simulink model "simulink_control"  (R2020b)
settings: Solver=FixedStepAuto  StartTime=0.0  StopTime=UI.motion_duration  FixedStep=UI.timestep  RelTol=1e-3
model workspace (MAT data in the model file):
  SL_ROS_VariableLengthArrays_MaxSizes.CommonInfo.ArrayTruncateAction = 'EmitWarning'
  SL_ROS_VariableLengthArrays_MaxSizes.MsgTypeMap = containers.Map
  SL_ROS_VariableLengthArrays_MaxSizes.MsgTypeMap.serialization.keys = {'ros_panda/JointCommandPosition'}
  SL_ROS_VariableLengthArrays_MaxSizes.MsgTypeMap.serialization.values{1}.PropertyName = 'Values'
  SL_ROS_VariableLengthArrays_MaxSizes.MsgTypeMap.serialization.values{1}.DataType = 'double'
  SL_ROS_VariableLengthArrays_MaxSizes.MsgTypeMap.serialization.values{1}.MaxLength = 7
  SL_ROS_VariableLengthArrays_MaxSizes.MsgTypeMap.serialization.uniformity = 0
  SL_ROS_VariableLengthArrays_MaxSizes.MsgTypeMap.serialization.keyType = 'char'
  SL_ROS_VariableLengthArrays_MaxSizes.MsgTypeMap.serialization.valueType = 'any'
values from neighbouring files (symbols this model uses):
  UI = []    [run_this_first.m]
undefined symbols (not defined in the file or in its folder): Stamp, Values, Values_SL_Info
libraries: robotlib x4
settings Model: ExtModeTrigDuration=40001  Creator=mojo  LastModifiedBy=mojo
settings OptimizationCC: EnhancedBackFolding=on  PassReuseOutputArgsAs=Individual arguments  ZeroExternalMemoryAtStartup=off  ZeroInternalMemoryAtStartup=off  MaxStackSize=64  OptimizeBlockOrder=speed  DifferentSizesBufferReuse=on  OptimizationCustomize=off  EfficientTunableParamExpr=on
settings DebuggingCC: ParameterTunabilityLossMsg=error
settings HardwareCC: ProdBitPerPointer=32  ProdBitPerSizeT=32  ProdBitPerPtrDiffT=32  ProdLargestAtomicFloat=None  ProdIntDivRoundTo=Undefined  ProdEndianess=Unspecified  ProdWordSize=32  ProdHWDeviceType=Generic->Unspecified (assume 32-bit Generic)
settings SFSimCC: MATLABDynamicMemAlloc=off
settings RTWCC: Description=Embedded Coder  SystemTargetFile=ert.tlc  HardwareBoard=Robot Operating System (ROS)  TLCOptions="-aInlineSetEventsForThisBaseRateFcn=TLC_FALSE -aSuppressMultiTaskScheduler=TLC_FALSE  -aRateBasedStepFcn=0"  TemplateMakefile=ert_default_tmf  Toolchain=Catkin  TargetLang=C++
settings CodeAppCC: ForceParamTrailComments=on  IgnoreCustomStorageClasses=off  OperatorAnnotations=on  SimulinkDataObjDesc=on  SFDataObjDesc=on  InsertBlockDesc=on

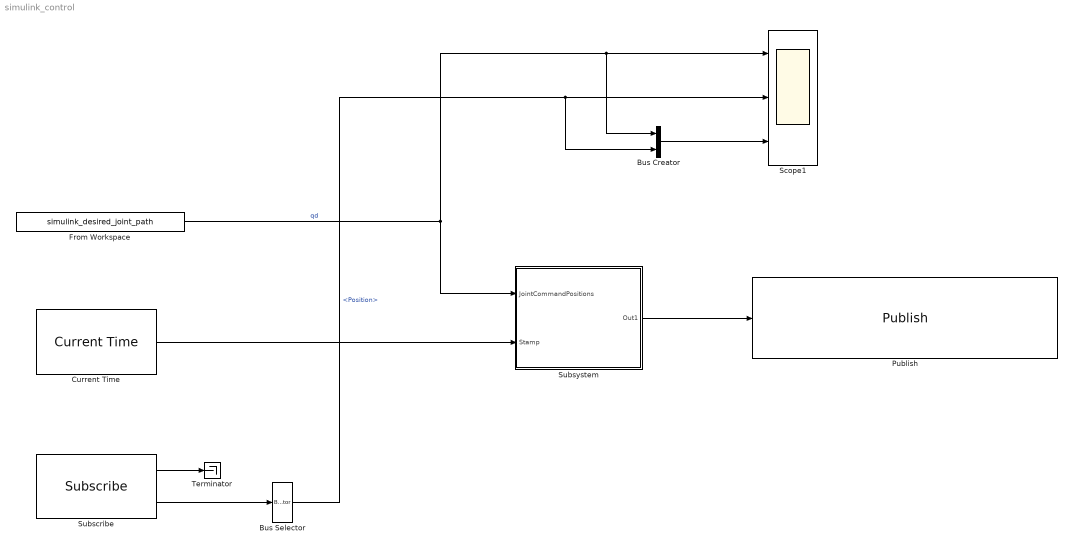
== system simulink_control ==
  Bus Creator : BusCreator  Inputs=2
  Bus Selector : BusSelector  OutputSignals=Position
  Current Time : robotlib/Current Time  OutputFormat=bus  SampleTime=-1  ModelName=simulink_control
      settings: SourceProductBaseCode=RR
  From Workspace : FromWorkspace  VariableName=simulink_desired_joint_path  SampleTime=UI.timestep
  Publish : robotlib/Publish  topicSource=Specify your own  topic=/franka_ros_interface/motion_controller/arm/joint_commands  messageType=franka_core_msgs/JointCommand  legacyBusStruct=off  messageQueueLength=1
  Scope1 : Scope  NumInputPorts=3
  Subscribe : robotlib/Subscribe  topicSource=Select from ROS network  topic=/joint_states  messageType=sensor_msgs/JointState  SampleTime=-1  legacyBusStruct=off  messageQueueLength=1
  Subsystem : Subsystem
  Terminator : Terminator
  wires:
  Current Time/1 -> Subsystem/2(Stamp)
  From Workspace/1 -> Bus Creator/1, Scope1/1, Subsystem/1(JointCommandPositions)  "qd"
  Subsystem/1(Out1) -> Publish/1
  Subscribe/1 -> Terminator/1
  Subscribe/2 -> Bus Selector/1
  Bus Creator/1 -> Scope1/3
  Bus Selector/1 -> Bus Creator/2, Scope1/2  "<Position>"

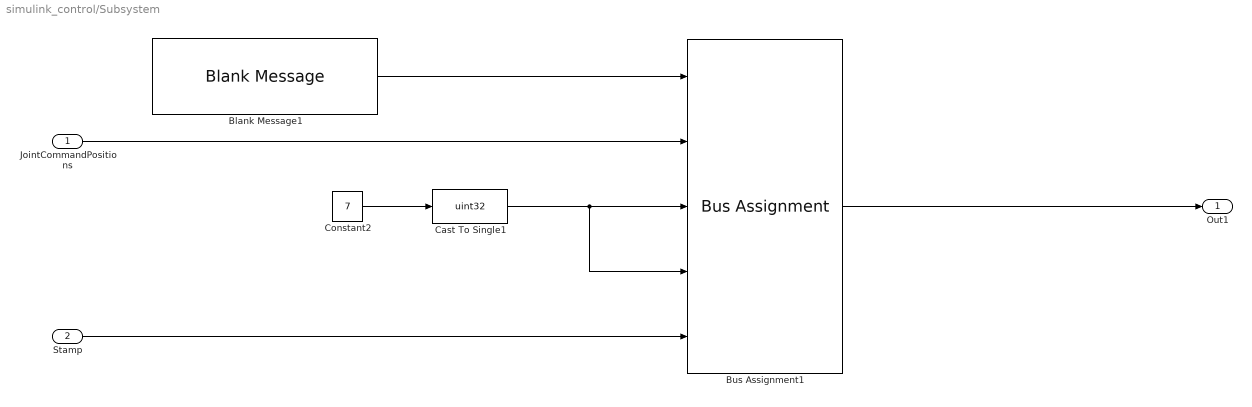
== system simulink_control/Subsystem ==
  JointCommandPositions : Inport
  Stamp : Inport  Port=2
  Blank Message1 : robotlib/Blank Message  messageClass=Message  entityType=franka_core_msgs/JointCommand  messageType=franka_core_msgs/JointCommand  SampleTime=inf  legacyBusStruct=off
  Bus Assignment1 : BusAssignment  AssignedSignals=Values,Values_SL_Info.CurrentLength,Values_SL_Info.ReceivedLength,Stamp
  Cast To Single1 : DataTypeConversion  OutDataTypeStr=uint32
  Constant2 : Constant  Value=7
  Out1 : Outport
  wires:
  Constant2/1 -> Cast To Single1/1
  JointCommandPositions/1 -> Bus Assignment1/2
  Cast To Single1/1 -> Bus Assignment1/4, Bus Assignment1/3
  Blank Message1/1 -> Bus Assignment1/1
  Stamp/1 -> Bus Assignment1/5
  Bus Assignment1/1 -> Out1/1
